simulink model "controller"  (R2024b)
settings: Solver=FixedStepAuto  StartTime=0.0  StopTime=10.0  FixedStep=1/100  RelTol=1e-3
undefined symbols (not defined in the file): MAX_RDB_ENGAGE_SPEED, MAX_TORQUE, MAX_TORQUE_REVERSE
settings Model: Creator=DAUIN-Win10  LastModifiedBy=aayan
settings OptimizationCC: ReuseModelBlockBuffer=off
settings DebuggingCC: UnconnectedInputMsg=warning  UnconnectedOutputMsg=warning  UnconnectedLineMsg=warning
settings ModelReferenceCC: EnableRefExpFcnMdlSchedulingChecks=on
settings RTWCC: GPUComputeCapability=3.5  DLArmComputeVersion=19.05

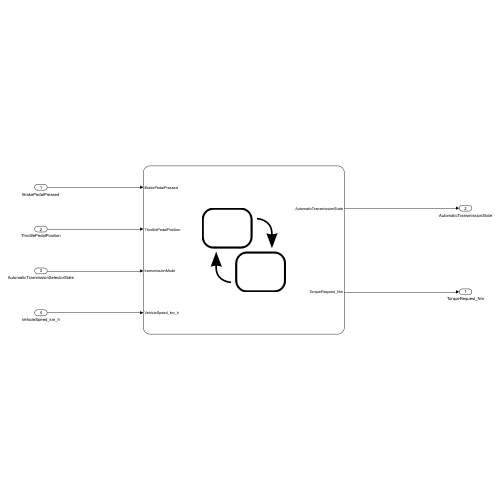
[thumbnail: Simulink's stored preview of the top-level diagram]
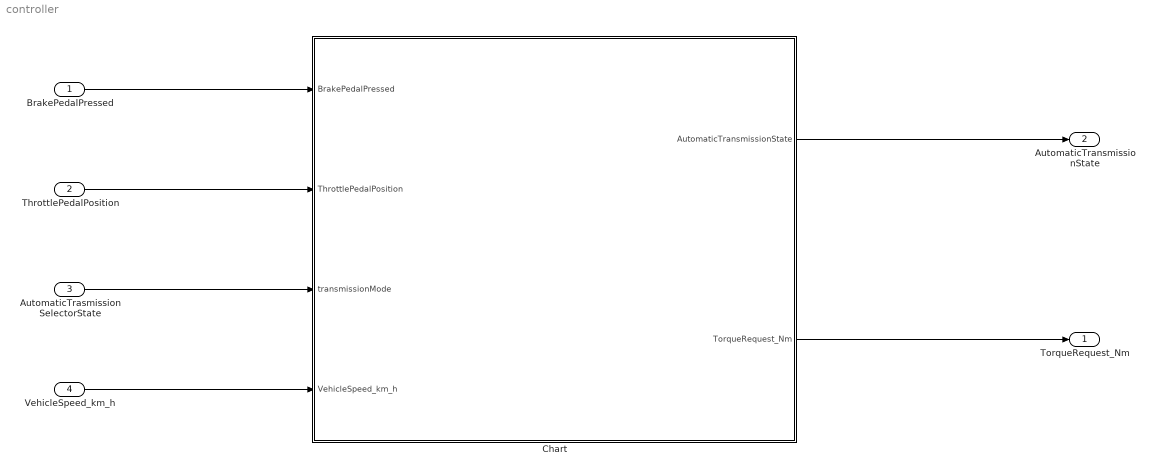
== system controller ==
  BrakePedalPressed : Inport  OutDataTypeStr=boolean
  ThrottlePedalPosition : Inport  Port=2  OutDataTypeStr=single
  AutomaticTrasmissionSelectorState : Inport  Port=3  OutDataTypeStr=Enum: TransmissionState
  VehicleSpeed_km_h : Inport  Port=4  OutDataTypeStr=single  Unit=km/h
  Chart : Stateflow chart  TreatAsAtomicUnit=on
  TorqueRequest_Nm : Outport  OutDataTypeStr=single  Unit=N*m
  AutomaticTransmissionState : Outport  Port=2  OutDataTypeStr=Enum: TransmissionState
  wires:
  BrakePedalPressed/1 -> Chart/1(BrakePedalPressed)
  ThrottlePedalPosition/1 -> Chart/2(ThrottlePedalPosition)
  AutomaticTrasmissionSelectorState/1 -> Chart/3(transmissionMode)
  VehicleSpeed_km_h/1 -> Chart/4(VehicleSpeed_km_h)
  Chart/1(AutomaticTransmissionState) -> AutomaticTransmissionState/1
  Chart/2(TorqueRequest_Nm) -> TorqueRequest_Nm/1

== stateflow chart controller/Chart ==
  state Park
    en:
    AutomaticTransmissionState = TransmissionState.Park;
    du:
    TorqueRequest_Nm = single(0);
  state Neutral
    en:
    AutomaticTransmissionState = TransmissionState.Neutral;
    du:
    TorqueRequest_Nm = single(0);
  state Drive
    en:
    AutomaticTransmissionState = TransmissionState.Drive;
    state ZeroTorque1
      du:
      TorqueRequest_Nm = single(0);
    state Acceleration
      du:
      TorqueRequest_Nm = single(MAX_TORQUE*(ThrottlePedalPosition));
    state StartToMove
      du:
      TorqueRequest_Nm = single(5);
    (default) -> ZeroTorque1
    ZeroTorque1 -> (junction 99) [order 1] : [BrakePedalPressed ~= 1 && VehicleSpeed_km_h  < 5 ]
    (junction 99) -> StartToMove
    (junction 94) -> ZeroTorque1
    StartToMove -> (junction 94) [order 2] : [BrakePedalPressed == 1]
    ZeroTorque1 -> Acceleration [order 2] : [(BrakePedalPressed ~= 1)]
    Acceleration -> ZeroTorque1 : [ (BrakePedalPressed == 1)]
    StartToMove -> Acceleration [order 1] : [ThrottlePedalPosition > 0 && BrakePedalPressed ~= 1]
  state Brake
    en:
    AutomaticTransmissionState = TransmissionState.Brake
    state AccelerationRegion
      du:
      TorqueRequest_Nm = single(MAX_TORQUE*(3/2)*(ThrottlePedalPosition - (1/3)));
    state ZeroTorque
      TorqueRequest_Nm = single(0);
    state DecelerationRegion
      du:
      TorqueRequest_Nm = single(-MAX_TORQUE*(1 - 3*ThrottlePedalPosition));
    (default) -> AccelerationRegion
    Brake.ZeroTorque -> AccelerationRegion : [ThrottlePedalPosition > (1/3) && BrakePedalPressed ~= 1]
    DecelerationRegion -> AccelerationRegion [order 1] : [ (ThrottlePedalPosition >(1/3)) && BrakePedalPressed ~= 1]
    AccelerationRegion -> DecelerationRegion : [ ThrottlePedalPosition < (1/3) ]
    (junction 43) -> Brake.ZeroTorque
    DecelerationRegion -> (junction 43) [order 2] : [VehicleSpeed_km_h < MAX_RDB_ENGAGE_SPEED]
  state Reverse
    en:
    AutomaticTransmissionState = TransmissionState.Reverse;
    state Deceleration
      du:
      TorqueRequest_Nm = single(-MAX_TORQUE_REVERSE*(ThrottlePedalPosition));
    state ZeroTorque
      TorqueRequest_Nm = single(0);
    (default) -> Deceleration
    Reverse.ZeroTorque -> Deceleration : [(BrakePedalPressed == 0)]
    Deceleration -> Reverse.ZeroTorque : [(BrakePedalPressed == 1)]
  (default) -> Park
  Neutral -> Drive [order 1] : [(BrakePedalPressed == 1) && (VehicleSpeed_km_h > -5) && ((transmissionMode == TransmissionState.Drive) || (transmissionMode == TransmissionState.Brake))]
  Park -> Neutral : [(BrakePedalPressed == 1) && (transmissionMode ~= TransmissionState.Park)]
  Drive -> Brake [order 1] : [ThrottlePedalPosition > (1/3) && (transmissionMode == TransmissionState.Brake)]
  Brake -> Drive : [ transmissionMode ~= TransmissionState.Brake]
  Drive -> Neutral [order 2] : [(transmissionMode ~= TransmissionState.Drive) && (transmissionMode ~= TransmissionState.Brake)]
  Neutral -> Park [order 3] : [(BrakePedalPressed == 1) && (abs(VehicleSpeed_km_h) <5) && transmissionMode == TransmissionState.Park]
  Neutral -> Reverse [order 2] : [(BrakePedalPressed == 1) && (VehicleSpeed_km_h < 5) && transmissionMode == TransmissionState.Reverse]
  Reverse -> Neutral : [transmissionMode ~= TransmissionState.Reverse]
  data: BrakePedalPressed input; ThrottlePedalPosition input; transmissionMode input; VehicleSpeed_km_h input; AutomaticTransmissionState output; TorqueRequest_Nm output; MAX_TORQUE parameter; MAX_TORQUE_REVERSE parameter; MAX_RDB_ENGAGE_SPEED parameter
